simulink model "subscriber_task"  (Simulink 3.0)
undefined symbols (not defined in the file): Double, F64
libraries: mathlib x4, mqttlib x2, arclib x2, stringlib x1

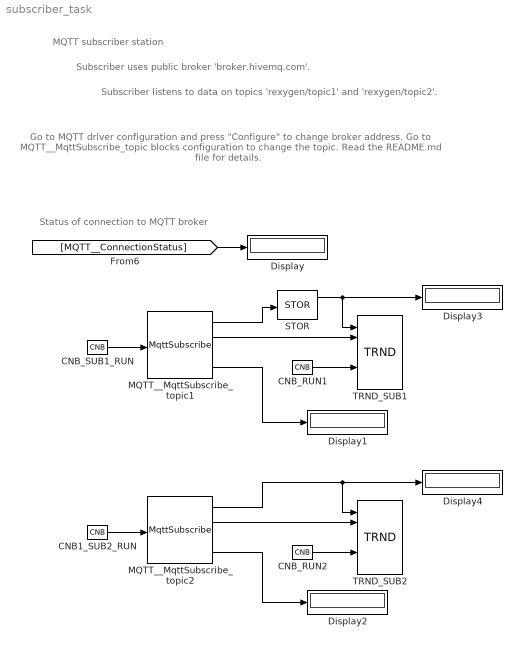
== system subscriber_task ==
  note: MQTT subscriber station
  note: Subscriber uses public broker 'broker.hivemq.com'.
  note: Subscriber listens to data on topics 'rexygen/topic1' and 'rexygen/topic2'.
  note: Status of connection to MQTT broker
  note: Go to MQTT driver configuration and press "Configure" to change broker address.
      | Go to MQTT__MqttSubscribe_topic blocks configuration to change the topic.
      |
      | Read the README.md file for details.
  CNB1_SUB2_RUN : mathlib/CNB  YCN=on
  CNB_RUN1 : mathlib/CNB  YCN=on
  CNB_RUN2 : mathlib/CNB  YCN=on
  CNB_SUB1_RUN : mathlib/CNB  YCN=on
  Display{,1..4} (5 alike) : Display
      Display settings: Format=Best fit
      Display1 settings: Format=Best fit
      Display2 settings: Format=Best fit
      Display3 settings: Format=short
      Display4 settings: Format=short
  MQTT__MqttSubscribe_topic1 : mqttlib/MqttSubscribe  topic=rexygen/topic1  QoS=1: QoS0 (At most once)  type=1: string  mode=1: Last value  defBuffSize=2048
  MQTT__MqttSubscribe_topic2 : mqttlib/MqttSubscribe  topic=rexygen/topic2  QoS=1: QoS0 (At most once)  type=2: double  mode=1: Last value  defBuffSize=2048
  STOR : stringlib/STOR  yerr=0
  TRND_SUB1 : arclib/TRND  n=4  l=1000  btype=8: Double (F64)  ptype1=1: Store  ptype2=1: Store  ptype3=1: Store  ptype4=1: Store  pfac=1  afac=0  arc=0  id=0  Title=Trend Title  timesrc=1: CORETIMER
  TRND_SUB2 : arclib/TRND  n=4  l=1000  btype=8: Double (F64)  ptype1=1: Store  ptype2=1: Store  ptype3=1: Store  ptype4=1: Store  pfac=1  afac=0  arc=0  id=0  Title=Trend Title  timesrc=1: CORETIMER
  wires:
  CNB1_SUB2_RUN/1 -> MQTT__MqttSubscribe_topic2/1
  CNB_RUN1/1 -> TRND_SUB1/5
  CNB_RUN2/1 -> TRND_SUB2/5
  CNB_SUB1_RUN/1 -> MQTT__MqttSubscribe_topic1/1
  [MQTT__ConnectionStatus] -> Display/1
  MQTT__MqttSubscribe_topic1/1 -> STOR/1
  MQTT__MqttSubscribe_topic1/2 -> TRND_SUB1/2
  MQTT__MqttSubscribe_topic1/4 -> Display1/1
  MQTT__MqttSubscribe_topic2/1 -> Display4/1, TRND_SUB2/1
  MQTT__MqttSubscribe_topic2/2 -> TRND_SUB2/2
  MQTT__MqttSubscribe_topic2/4 -> Display2/1
  STOR/1 -> Display3/1, TRND_SUB1/1
